simulink model "scenario_sensor_model"  (R2026a)
settings: Solver=VariableStepAuto
undefined symbols (not defined in the file or in its folder): driving, sock
libraries: drivingscenarioandsensors x2
settings Model: Creator=user  LastModifiedBy=user

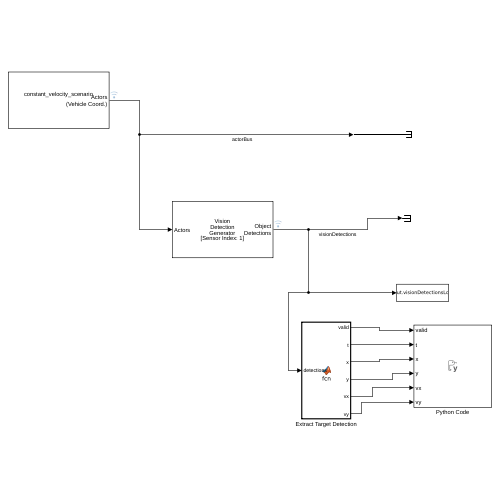
[thumbnail: Simulink's stored preview of the top-level diagram]
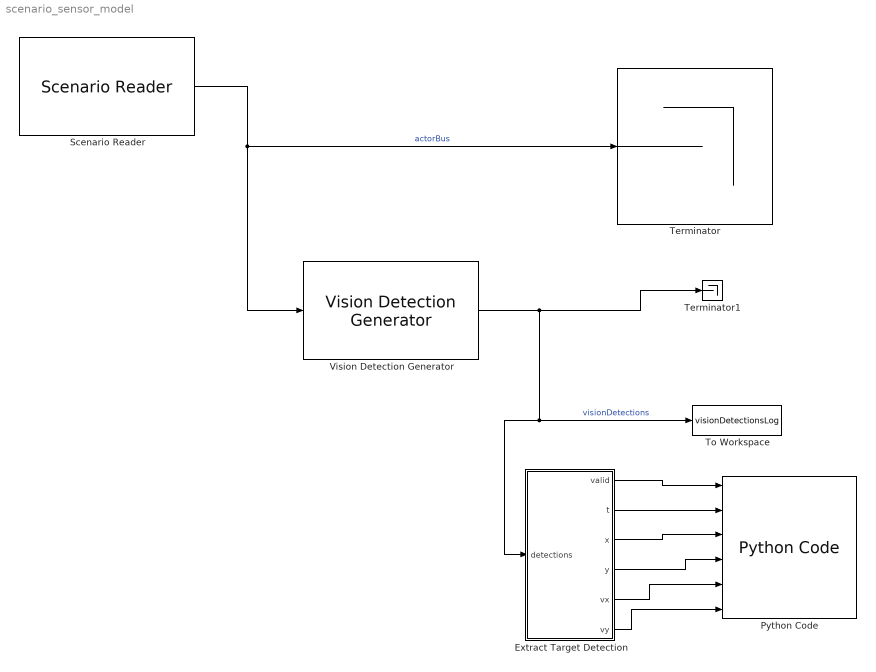
== system scenario_sensor_model ==
  Extract Target Detection : MATLAB Function  TreatAsAtomicUnit=on
  Python Code : PythonCode  InitializeConditionsCode=|  OutputCode=|  TerminateCode=sock.close()  SampleTime=0.1
      InitializeConditionsCode=|
      | import socket
      | 
      | sock = socket.socket(socket.AF_INET, socket.SOCK_DGRAM)
      OutputCode=|
      | import struct
      | 
      | if bool(valid):
      |     payload = struct.pack(
      |         "<5d",
      |         float(t),
      |         float(x),
      |         float(y),
      |         float(vx),
      |         float(vy)
      |     )
      | 
      |     sock.sendto(payload, ("127.0.0.1", 51001))
  Scenario Reader : drivingscenarioandsensors/Scenario Reader  ScenarioSource=From file  ScenarioFileName=/home/user/Desktop/latency-aware-target-control/simulation/simulink/constant_velocity_scenario.mat  ScenarioVariableName=scenario  OutputCoordinateSystem=Vehicle coordinates  EgoVehicleSource=Scenario  EgoVehicleActorID=1  OrientVehiclesOnRoad=off  OutputEgoVehiclePose=off  OutputEgoVehicleState=off  SampleTime=0.1  LaneBoundaryOutput=None  LaneBoundaryDistance=0:0.5:9.5  LaneBoundaryLocation=Center of lane markings  BusNameSource=Auto  BusName=BusActors  BusNumActorsSource=Scenario  BusNumActors=100  BusName2Source=Auto  BusName2=BusLaneBoundaries  BusNumLaneBoundariesSource=Scenario  BusNumLaneBoundaries=10  BusName3Source=Auto  BusName3=BusEgoActor  BusName4Source=Auto  BusName4=BusEgoState  ShowCoordinateLabels=on  SimulateUsing=Interpreted execution
  Terminator : Terminator
  Terminator1 : Terminator
  To Workspace : ToWorkspace  VariableName=visionDetectionsLog  SaveFormat=Timeseries  SampleTime=-1
  Vision Detection Generator : drivingscenarioandsensors/Vision Detection Generator  SensorIndex=1  DetectorOutput=Objects only  UpdateInterval=0.1  LaneUpdateInterval=0.1  SensorLocation=[ 1.9, 0 ]  Height=1.1  Yaw=0  Pitch=1  Roll=0  BusNameSource=Auto  BusName=BusObjectDetections  BusName2Source=Auto  BusName2=BusLaneDetections  MaxNumDetectionsSource=Property  MaxNumDetections=50  MaxNumLanesSource=Property  MaxNumLanes=30  DetectionCoordinates=Ego Cartesian  SimulateUsing=Interpreted execution  MaxRange=150  BoundingBoxAccuracy=5  ProcessNoiseIntensity=5  MaxSpeed=100  MaxAllowedOcclusion=0.5  MinObjectImageSize=[ 15, 15 ]  DetectionProbability=0.7  FalsePositivesPerImage=1.0  MinLaneImageSize=[ 20, 3 ]  LaneBoundaryAccuracy=3  HasNoise=on  InitialSeedSource=Specify seed  InitialSeed=42  UsedSeed=driving.internal.SimulinkUtilities.seedManager(gcb)  ActorProfilesSource=From Scenario Reader block  ActorProfilesParameters=driving.internal.ActorProfilesParameters  ActorProfilesExpression=struct( 'ClassID', 0, 'Length', 4.7, 'Width', 1.8, 'Height', 1.4, 'OriginOffset', [ -1.35, 0, 0 ] )  Intrinsics=driving.internal.cameraIntrinsics
  wires:
  Scenario Reader/1 -> Vision Detection Generator/1, Terminator/1  "actorBus"
  Vision Detection Generator/1 -> Terminator1/1, Extract Target Detection/1(detections), To Workspace/1  "visionDetections"
  Extract Target Detection/2(t) -> Python Code/2
  Extract Target Detection/3(x) -> Python Code/3
  Extract Target Detection/4(y) -> Python Code/4
  Extract Target Detection/5(vx) -> Python Code/5
  Extract Target Detection/6(vy) -> Python Code/6
  Extract Target Detection/1(valid) -> Python Code/1

== matlab function scenario_sensor_model/Extract Target Detection ==
  data: valid output; t output; x output; detections input; y output; vx output; vy output
function [valid, t, x, y, vx, vy] = fcn(detections)

targetActorId = 2;

% Default outputs
valid = false;

t  = 0.0;
x  = 0.0;
y  = 0.0;
vx = 0.0;
vy = 0.0;

% Sensor did not generate a valid update at this step.
if ~detections.IsValidTime
    return;
end

n = detections.NumDetections;

for detectionIdx = 1:n

    targetIndex = ...
        detections.Detections(detectionIdx) ...
        .ObjectAttributes.TargetIndex;

    % False positives and other actors are ignored.
    if targetIndex ~= targetActorId
        continue;
    end

    measurement = ...
        detections.Detections(detectionIdx).Measurement;

    t = detections.Detections(detectionIdx).Time;

    x  = measurement(1);
    y  = measurement(2);
    vx = measurement(4);
    vy = measurement(5);

    valid = true;

    % Only one target vehicle is required.
    return;
end
